simulink model "syncbuck_OL"  (Simulink 7.5)
settings: Solver=ode45  StartTime=0.0  StopTime=100e-6  MaxStep=0.1e-6  RelTol=1e-3
libraries: simulink x1
settings Model: Creator=Dragan Maksimovic  LastModifiedBy=Dragan Maksimovic

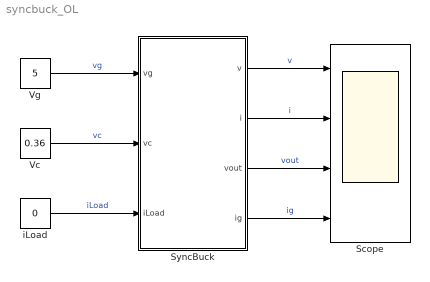
== system syncbuck_OL ==
  Scope : Scope  NumInputPorts=4
      settings: YMin=-5~-5~-5~-5  YMax=5~5~5~5
  SyncBuck : Subsystem  mask{L=1e-6, i0=0, C=200e-6, v0=1.8, fs=1e6, VM=1, Ron1=20e-3, Ron2=20e-3, RL=10e-3, Resr=0.8e-3, sw=off}
      mask prompts: L "Inductance L"; i0 "Initial inductor current i(0)"; C "Capacitance C"; v0 "Initial capacitor voltage v(0)"; fs "Switching frequency fs"; VM "PWM ramp amplitude VM"; Ron1 "Transistor switch Ron1"; Ron2 "Sync rectifier switch Ron2"; RL "Inductor resistance RL"; Resr "Capacitor esr Resr"; sw "Switching model?"
  Vc : Constant  Value=0.36  OutDataType=fixdt(1, 16)  OutScaling=2^0
  Vg : Constant  Value=5  OutDataType=fixdt(1, 16)  OutScaling=2^0
  iLoad : Constant  Value=0  OutDataType=fixdt(1, 16)  OutScaling=2^0
  wires:
  Vg/1 -> SyncBuck/1(vg)  "vg"
  Vc/1 -> SyncBuck/2(vc)  "vc"
  iLoad/1 -> SyncBuck/3(iLoad)  "iLoad"
  SyncBuck/1(v) -> Scope/1  "v"
  SyncBuck/2(i) -> Scope/2  "i"
  SyncBuck/3(vout) -> Scope/3  "vout"
  SyncBuck/4(ig) -> Scope/4  "ig"

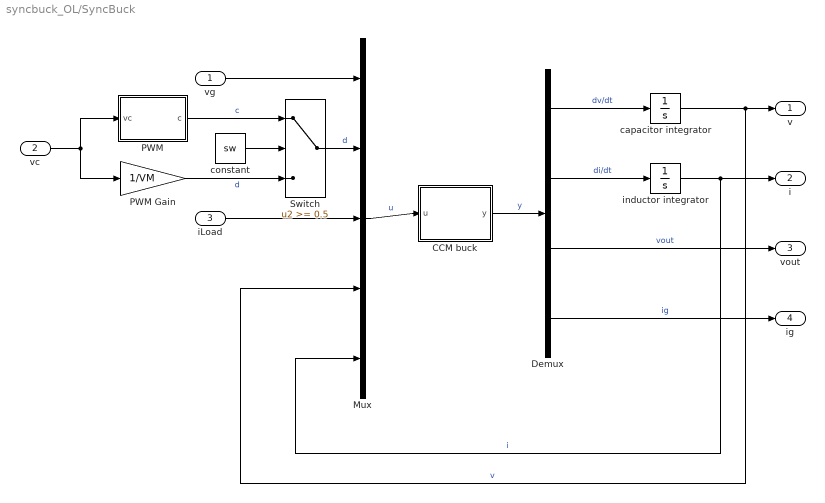
== system syncbuck_OL/SyncBuck ==
  vg : Inport  OutDataType=fixdt(1, 16)  OutScaling=2^0
  vc : Inport  Port=2  OutDataType=fixdt(1, 16)  OutScaling=2^0
  iLoad : Inport  Port=3  OutDataType=fixdt(1, 16)  OutScaling=2^0
  CCM buck : Stateflow chart  TreatAsAtomicUnit=on
  Demux : Demux
  Mux : Mux  Inputs=5
  PWM : Subsystem
  PWM Gain : Gain  Gain=1/VM  ParameterDataType=fixdt(1, 16)  ParameterScaling=2^0  OutDataType=fixdt(1, 16)  OutScaling=2^0
  Switch : Switch  Threshold=0.5  OutDataType=fixdt(1, 16)  OutScaling=2^0
  capacitor integrator : Integrator  InitialCondition=v0
  constant : Constant  Value=sw  OutDataType=fixdt(1, 16)  OutScaling=2^0
  inductor integrator : Integrator  InitialCondition=i0
  v : Outport  OutDataType=fixdt(1, 16)  OutScaling=2^0
  i : Outport  Port=2  OutDataType=fixdt(1, 16)  OutScaling=2^0
  vout : Outport  Port=3  OutDataType=fixdt(1, 16)  OutScaling=2^0
  ig : Outport  Port=4  OutDataType=fixdt(1, 16)  OutScaling=2^0
  wires:
  Demux/1 -> capacitor integrator/1  "dv/dt"
  capacitor integrator/1 -> v/1, Mux/4  "v"
  inductor integrator/1 -> i/1, Mux/5  "i"
  Demux/2 -> inductor integrator/1  "di/dt"
  Demux/3 -> vout/1  "vout"
  Demux/4 -> ig/1  "ig"
  CCM buck/1(y) -> Demux/1  "y"
  vg/1 -> Mux/1
  iLoad/1 -> Mux/3
  Mux/1 -> CCM buck/1(u)  "u"
  Switch/1 -> Mux/2  "d"
  constant/1 -> Switch/2
  vc/1 -> PWM/1(vc), PWM Gain/1
  PWM/1(c) -> Switch/1  "c"
  PWM Gain/1 -> Switch/3  "d"

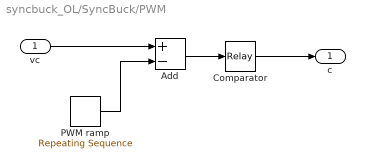
== system syncbuck_OL/SyncBuck/PWM ==
  vc : Inport  OutDataType=fixdt(1, 16)  OutScaling=2^0
  Add : Sum  Inputs=+-  OutDataType=fixdt(1, 16)  OutScaling=2^-10
  Comparator : Relay  OutDataType=fixdt(1, 16)  OutScaling=2^0
  PWM ramp : simulink/Sources/Repeating Sequence  SystemSampleTime=-1  rep_seq_t=[0 1/fs]  rep_seq_y=[0 VM]
  c : Outport  OutDataType=fixdt(1, 16)  OutScaling=2^0
  wires:
  vc/1 -> Add/1
  PWM ramp/1 -> Add/2
  Add/1 -> Comparator/1
  Comparator/1 -> c/1

== matlab function SyncBuck/CCM buck ==
  data: u input double size=5; y output double; L parameter double; C parameter double; RL parameter double; Ron1 parameter double; Ron2 parameter double; Resr parameter double
function y = CCMbuck(u,L,C,RL,Ron1,Ron2,Resr)
% State equations of a synchronous buck converter
% Conduction losses due to RL, Ron1, Ron2, Resr are included
% Inputs: u = [vg d iLoad v i]
% Outputs: y = [iC/C vL/L vout ig]
% Parameters: L, C, RL, Ron1, Ron2, Resr
%
% variables
vg = u(1); % input voltage
d = u(2); % switch control d=c (in the switching model), d in the averaged model
iLoad = u(3); % load current
v = u(4); % capacitor voltage
i = u(5); % inductor current
%
% state equations
vout = v + Resr*(i-iLoad); % output voltage
ig = d*i; % input current
iC = i - iLoad; % capacitor current
vL = d*(vg-(Ron1+RL)*i-vout)+(1-d)*(-(Ron2+RL)*i - vout); % inductor voltage
%
% output
y = [iC/C vL/L vout ig];
